simulink model "mCSControls_DG"  (R2012b)
settings: Solver=FixedStepDiscrete  StartTime=0.0  StopTime=10.0  RelTol=1e-3
values from neighbouring files (symbols this model uses):
  CDF2FThreshold = 45    [ControlCal_DG.m]
  CDF2TempThreshold = 20    [ControlCal_DG.m]
  delay = 5    [ControlCal_DG.m]
  DFThresh = 33    [ControlCal_DG.m]
  H = [90 90 90 90]    [ControlCal_DG.m]
  HeatTempThresh1 = 40    [ControlCal_DG.m]
  HeatTempThresh2 = 30    [ControlCal_DG.m]
  HeatTempThresh3 = 20    [ControlCal_DG.m]
  HStabilizationTime = 2*60    (= 120)    [ControlCal_DG.m]
  I_FAN = -1    [ControlCal_DG.m]
  I_VALVE = -1    [ControlCal_DG.m]
  initialSet = [1 1 1]    [ControlCal_DG.m]
  PBFTempThreshold = 30    [ControlCal_DG.m]
  PowerModeSwitchDelay = 30    [ControlCal_DG.m]
  SVocThresh = 550    [ControlCal_DG.m]
  T = [0 4 7 10]    [ControlCal_DG.m]
  Ts = 0.5    [ControlCal_DG.m]
  TSTempSetPoint = -2    [ControlCal_DG.m]
  TV1FThresh = 45    [ControlCal_DG.m]
  TV2FThresh = 60    [ControlCal_DG.m]
  VbatThresh = 22    [ControlCal_DG.m]
  VocDecRate = 0.5    [ControlCal_DG.m]
  VocIncrement = 5    [ControlCal_DG.m]
libraries: c2833xlib x29, simulink x23, c280xlib x11, idelinklib_tgtpref x1
(part 1 of 4)
settings Model: Creator=vinay  LastModifiedBy=vinay
settings DataIOCC: SaveOutput=off  SaveTime=off
settings OptimizationCC: InlineParams=on  UseFloatMulNetSlope=on  UseSpecifiedMinMax=on  InlineInvariantSignals=on  EnhancedBackFolding=on  ZeroExternalMemoryAtStartup=off  NoFixptDivByZeroProtection=on  EfficientFloat2IntCast=on  OptimizeModelRefInitCode=on  LifeSpan=1
settings DebuggingCC: MultiTaskCondExecSysMsg=warning
settings HardwareCC: ProdBitPerChar=16  ProdBitPerInt=16  ProdBitPerPointer=16  ProdLargestAtomicInteger=Integer  ProdIntDivRoundTo=Zero  ProdEndianess=LittleEndian  ProdWordSize=16  ProdHWDeviceType=Texas Instruments->C2000
settings RTWCC: SystemTargetFile=idelink_ert.tlc  GenerateMakefile=off  TemplateMakefile=none  Description=IDE Link ERT  ProcessScript=idelink_ert_make_rtw_hook  CustomInclude=C:\X\DesignFiles\Controls\Gen2\CPUOverrunDetection\  CustomSource=C:\X\DesignFiles\Controls\Gen2\CPUOverrunDetection\CPUOverrunDetection.c  RTWCompilerOptimization=On
settings CodeAppCC: IgnoreCustomStorageClasses=off

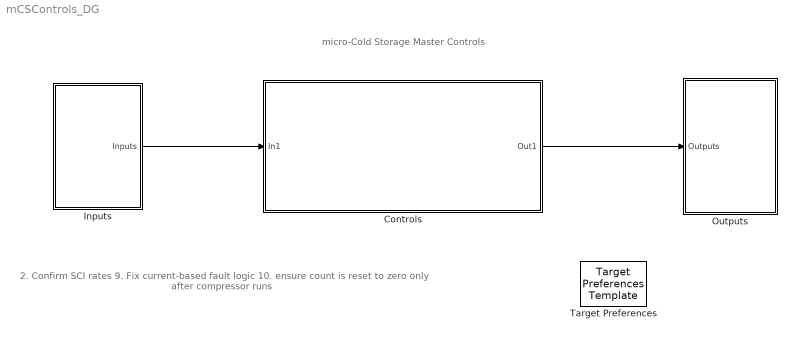
== system mCSControls_DG ==
  note: 2. Confirm SCI rates
      | 9. Fix current-based fault logic
      | 10. ensure count is reset to zero only after compressor runs
  note: micro-Cold Storage Master Controls
  Controls : Subsystem
  Inputs : Subsystem
  Outputs : Subsystem
  Target Preferences : idelinklib_tgtpref/Target Preferences Template  Tag=ccslinktgtpref_ccsv4  library=off
  wires:
  Inputs/1(Inputs) -> Controls/1(In1)
  Controls/1(Out1) -> Outputs/1(Outputs)

== system mCSControls_DG/Controls ==
  In1 : Inport
  Bus Creator : BusCreator  Inputs=2
  Chart : Stateflow chart  TreatAsAtomicUnit=on
  RelayInitialization : Subsystem
  Out1 : Outport
  wires:
  Bus Creator/1 -> Out1/1  "IO"
  In1/1 -> Chart/1(Inputs), Bus Creator/1
  RelayInitialization/1(Relays) -> Chart/2(RelaysOff)
  Chart/1(RelaysOP) -> Bus Creator/2

== system mCSControls_DG/Inputs ==
  Bus Creator : BusCreator  Inputs=6
  DCParams_And_Sensors : Subsystem
  DriveParams : Subsystem
  EEPROM : Subsystem  Commented=on
  HMI : Subsystem
  PowerIP : Subsystem
  Inputs : Outport
  wires:
  Bus Creator/1 -> Inputs/1  "Inputs"
  DCParams_And_Sensors/1(DCParams) -> Bus Creator/1
  DCParams_And_Sensors/2(Sensors) -> Bus Creator/2
  DriveParams/1(DriveParams) -> Bus Creator/3
  HMI/1(HMI) -> Bus Creator/4
  EEPROM/1(EEPROM) -> Bus Creator/5
  PowerIP/1(PowerIP) -> Bus Creator/6

== system mCSControls_DG/Outputs ==
  Outputs : Inport
  DataLogger : Subsystem
  EEPROM : Subsystem  Commented=on
  LCD : Subsystem
  Relays : Subsystem
  wires:
  Outputs/1 -> Relays/1(Inputs), DataLogger/1(Inputs), LCD/1(Inputs), EEPROM/1(Inputs)

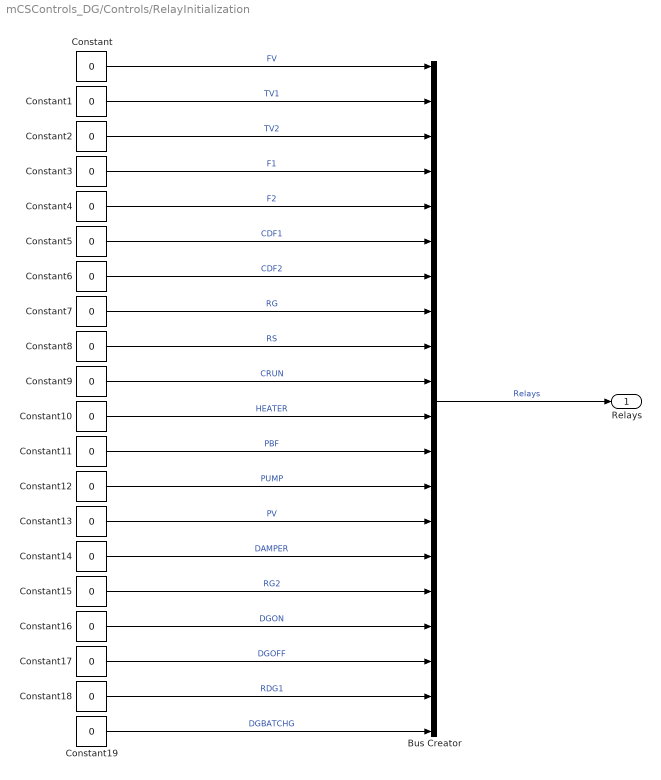
== system mCSControls_DG/Controls/RelayInitialization ==
  Bus Creator : BusCreator  Inputs=20
  Constant{,1..19} (20 alike) : Constant  Value=0  OutDataTypeStr=double
  Relays : Outport
  wires:
  Constant/1 -> Bus Creator/1  "FV"
  Constant13/1 -> Bus Creator/14  "PV"
  Constant12/1 -> Bus Creator/13  "PUMP"
  Constant11/1 -> Bus Creator/12  "PBF"
  Constant10/1 -> Bus Creator/11  "HEATER"
  Constant9/1 -> Bus Creator/10  "CRUN"
  Constant8/1 -> Bus Creator/9  "RS"
  Constant7/1 -> Bus Creator/8  "RG"
  Constant6/1 -> Bus Creator/7  "CDF2"
  Constant5/1 -> Bus Creator/6  "CDF1"
  Constant4/1 -> Bus Creator/5  "F2"
  Constant3/1 -> Bus Creator/4  "F1"
  Constant2/1 -> Bus Creator/3  "TV2"
  Constant1/1 -> Bus Creator/2  "TV1"
  Bus Creator/1 -> Relays/1  "Relays"
  Constant14/1 -> Bus Creator/15  "DAMPER"
  Constant15/1 -> Bus Creator/16  "RG2"
  Constant18/1 -> Bus Creator/19  "RDG1"
  Constant17/1 -> Bus Creator/18  "DGOFF"
  Constant16/1 -> Bus Creator/17  "DGON"
  Constant19/1 -> Bus Creator/20  "DGBATCHG"

== system mCSControls_DG/Inputs/DCParams_And_Sensors ==
  Bus Creator : BusCreator  Inputs=8
  Bus Creator1 : BusCreator  Inputs=9
  Data Type Conversion : DataTypeConversion  OutDataTypeStr=double
  SCI C : c280xlib/SCI Receive  sciModule=C  dataHead=''  dataTail=''  dataType=int16  dataDim=8  initValue=0  errOption=Output the last received value  errValue=0  sampleTime=Ts  outputStatus=off  postInterrupt=off  numFifo=1
  SignalSeperationAndMerging : Subsystem
  DCParams : Outport
  Sensors : Outport  Port=2
  wires:
  SignalSeperationAndMerging/1(Voc) -> Bus Creator/1  "Voc"
  SignalSeperationAndMerging/8(GRID) -> Bus Creator/8  "GRID"
  SignalSeperationAndMerging/2(VBat) -> Bus Creator/2  "Vbat"
  SignalSeperationAndMerging/3(ILoad) -> Bus Creator/3  "Iload"
  SignalSeperationAndMerging/4(IString) -> Bus Creator/4  "Istring"
  SignalSeperationAndMerging/5(F1_HPS) -> Bus Creator/5  "F1_HPS"
  SignalSeperationAndMerging/6(F2_LPS) -> Bus Creator/6  "F2_LPS"
  SignalSeperationAndMerging/7(F3_INT69) -> Bus Creator/7  "F3_INT69"
  Bus Creator/1 -> DCParams/1  "DCParams"
  Bus Creator1/1 -> Sensors/1  "Sensors"
  Data Type Conversion/1 -> SignalSeperationAndMerging/1(Data)
  SignalSeperationAndMerging/9(TH1) -> Bus Creator1/1  "TH1"
  SignalSeperationAndMerging/10(TA) -> Bus Creator1/2  "TA"
  SignalSeperationAndMerging/11(TES1) -> Bus Creator1/3  "TES1"
  SignalSeperationAndMerging/12(TES2) -> Bus Creator1/4  "TES2"
  SignalSeperationAndMerging/13(RH1) -> Bus Creator1/5  "RH1"
  SignalSeperationAndMerging/14(RA) -> Bus Creator1/6  "RA"
  SignalSeperationAndMerging/15(Door) -> Bus Creator1/7  "Door"
  SignalSeperationAndMerging/16(Tank) -> Bus Creator1/8  "Tank"
  SCI C/1 -> Data Type Conversion/1
  SignalSeperationAndMerging/17(Pressure) -> Bus Creator1/9  "Pressure"

== system mCSControls_DG/Inputs/DriveParams ==
  Bus Creator : BusCreator  Inputs=1
  Bus Creator1 : BusCreator  Inputs=3
  Bus Creator2 : BusCreator  Inputs=2
  Demux : Demux
  DriveParamReceive : Subsystem
  From : From  Commented=on  GotoTag=DriveFreq  TagVisibility=global
  Subsystem1 : Subsystem  Commented=on
  DriveParams : Outport
  wires:
  Demux/4 -> Bus Creator/1  "FAULTS"
  Demux/3 -> Bus Creator1/3  "OPCurr"
  Bus Creator1/1 -> Bus Creator2/1  "OP"
  Bus Creator/1 -> Bus Creator2/2  "FAULTS"
  Bus Creator2/1 -> DriveParams/1  "DriveParams"
  DriveParamReceive/1(Data) -> Demux/1
  Demux/1 -> Bus Creator1/1  "OPFreq"
  Demux/2 -> Bus Creator1/2  "OPPower"

== system mCSControls_DG/Inputs/EEPROM ==
  Bus Creator : BusCreator  Inputs=3
  Compare To Zero : simulink/Logic and Bit Operations/Compare To Zero  relop===  OutDataTypeStr=boolean
  Constant : Constant  Value=initialSet
  Data Type Conversion : DataTypeConversion  OutDataTypeStr=double
  Demux : Demux  Outputs=3
  EEPROMRead : Subsystem
  Rate Transition : RateTransition  X0=initialSet  OutPortSampleTime=Ts
  Rate Transition1 : RateTransition  Deterministic=off  OutPortSampleTime=Ts
  Terminator : Terminator
  EEPROM : Outport
  tag scope: Reading=global
  wires:
  Data Type Conversion/1 -> Demux/1
  Demux/1 -> Bus Creator/1  "B"
  Demux/2 -> Bus Creator/2  "M1"
  Demux/3 -> Bus Creator/3  "P1"
  Bus Creator/1 -> EEPROM/1  "EEPROM1"
  Rate Transition/1 -> Data Type Conversion/1
  [Writing] -> Compare To Zero/1
  Compare To Zero/1 -> EEPROMRead/Enable
  EEPROMRead/2(Reading) -> Rate Transition1/1
  Rate Transition1/1 -> [Reading]
  EEPROMRead/1(D) -> Terminator/1
  Constant/1 -> Rate Transition/1

== system mCSControls_DG/Inputs/HMI ==
  Bus Creator : BusCreator  Inputs=3
  Data Detection : MATLAB Function  TreatAsAtomicUnit=on
  Data Type Conversion : DataTypeConversion  OutDataTypeStr=double
  Memory : Memory  X0=initialSet(1)  InheritSampleTime=on
  Memory1 : Memory  X0=initialSet(2)  InheritSampleTime=on
  Memory2 : Memory  X0=initialSet(3)  InheritSampleTime=on
  Rate Transition : RateTransition  Deterministic=off  X0=[250 initialSet 250]
  SCI A Receive : Subsystem
  HMI : Outport
  wires:
  Data Detection/1(B) -> Memory/1, Bus Creator/1  "B"
  Data Detection/2(M1) -> Bus Creator/2, Memory1/1  "M1"
  Data Detection/3(P1) -> Memory2/1, Bus Creator/3  "P1"
  Bus Creator/1 -> HMI/1  "EEPROM"
  Data Type Conversion/1 -> Data Detection/1(u)
  [receiveTrigger] -> SCI A Receive/Trigger
  Memory/1 -> Data Detection/2(Bp)
  Memory1/1 -> Data Detection/3(M1p)
  Memory2/1 -> Data Detection/4(P1p)
  SCI A Receive/1(Out1) -> Rate Transition/1
  Rate Transition/1 -> Data Type Conversion/1

== system mCSControls_DG/Inputs/PowerIP ==
  Bus Creator : BusCreator  Inputs=1
  Constant : Constant  Commented=on
  Data Type Conversion : DataTypeConversion  OutDataTypeStr=double
  Digital Input : c2833xlib/Digital Input  GPIO_Number=GPIO0~GPIO7  GPIO_Bit0=off  GPIO_Bit1=off  GPIO_Bit2=off  GPIO_Bit3=off  GPIO_Bit4=off  GPIO_Bit5=on  GPIO_Bit6=off  GPIO_Bit7=off  sampleTime=Ts  dataType=int16  GPIO_Bit0_Qualification=Sync to SYSCLKOUT  GPIO_Bit1_Qualification=Sync to SYSCLKOUT  GPIO_Bit2_Qualification=Sync to SYSCLKOUT  GPIO_Bit3_Qualification=Sync to SYSCLKOUT  GPIO_Bit4_Qualification=Sync to SYSCLKOUT  GPIO_Bit5_Qualification=Sync to SYSCLKOUT  GPIO_Bit6_Qualification=Sync to SYSCLKOUT  GPIO_Bit7_Qualification=Sync to SYSCLKOUT  Qualification_Period=-1
  Terminator : Terminator  Commented=on
  PowerIP : Outport
  wires:
  Data Type Conversion/1 -> Bus Creator/1  "PowerIP"
  Bus Creator/1 -> PowerIP/1  "PowerIP"
  Digital Input/1 -> Data Type Conversion/1

== system mCSControls_DG/Outputs/DataLogger ==
  Inputs : Inport
  ASCIIAndDataPackaging : Subsystem
  Data Type Conversion1 : DataTypeConversion  Commented=on  OutDataTypeStr=uint8  RndMeth=Simplest
  Debugging : Subsystem  Commented=on
  Rate Transition1 : RateTransition  Deterministic=off  OutPortSampleTime=Tlog
  SCI C : c280xlib/SCI Transmit  sciModule=C  dataHead=''  dataTail=''  postInterrupt=off  numFifo=1
  SCI C1 : c280xlib/SCI Transmit  Commented=on  sciModule=C  dataHead=''  dataTail=''  postInterrupt=off  numFifo=1
  wires:
  ASCIIAndDataPackaging/1(Out1) -> SCI C/1
  Rate Transition1/1 -> ASCIIAndDataPackaging/1(In1)
  Debugging/1(Out1) -> Data Type Conversion1/1
  Data Type Conversion1/1 -> SCI C1/1
  Inputs/1 -> Debugging/1(GUIData), Rate Transition1/1

== system mCSControls_DG/Outputs/EEPROM ==
  Inputs : Inport
  Bus Selector1 : BusSelector  OutputSignals=Inputs.EEPROM  OutputAsBus=on
  ChangeDetection : Subsystem
  OneSecTimer : Stateflow chart  TreatAsAtomicUnit=on
  Subsystem : Subsystem
  tag scope: Writing=global
  wires:
  Inputs/1 -> Bus Selector1/1
  Bus Selector1/1 -> Subsystem/1(D), ChangeDetection/1(D)
  ChangeDetection/1(Change) -> OneSecTimer/1(Input)
  [Reading] -> OneSecTimer/2(Reading)
  OneSecTimer/1(Enable) -> Subsystem/Trigger, [Writing]

== system mCSControls_DG/Outputs/LCD ==
  Inputs : Inport
  Compare To Constant : simulink/Logic and Bit Operations/Compare To Constant  relop===  const=1  OutDataTypeStr=boolean
  Compare To Constant1 : simulink/Logic and Bit Operations/Compare To Constant  relop===  const=2  OutDataTypeStr=boolean
  Compare To Constant2 : simulink/Logic and Bit Operations/Compare To Constant  relop===  const=3  OutDataTypeStr=boolean
  Compare To Constant3 : simulink/Logic and Bit Operations/Compare To Constant  relop===  const=5  OutDataTypeStr=boolean
  DE_RE_One : Subsystem
  DE_RE_Zero : Subsystem
  Rate Transition : RateTransition
  Repeating Sequence Stair : simulink/Sources/Repeating Sequence Stair  OutValues=[1 2 3 4 5].'  tsamp=0.1  OutMin=[]  OutMax=[]  OutDataTypeStr=double  OutputDataTypeScalingMode=double  OutDataType=fixdt(0,8)  ConRadixGroup=Best Precision: Vector-wise  OutScaling=2^-12
  Transmit : Subsystem
  tag scope: receiveTrigger=global
  wires:
  Repeating Sequence Stair/1 -> Compare To Constant3/1, Compare To Constant2/1, Compare To Constant1/1, Compare To Constant/1
  Inputs/1 -> Rate Transition/1
  Compare To Constant2/1 -> DE_RE_Zero/Trigger
  Compare To Constant/1 -> DE_RE_One/Enable
  Compare To Constant1/1 -> Transmit/Trigger
  Rate Transition/1 -> Transmit/1(Inputs)
  Compare To Constant3/1 -> [receiveTrigger]

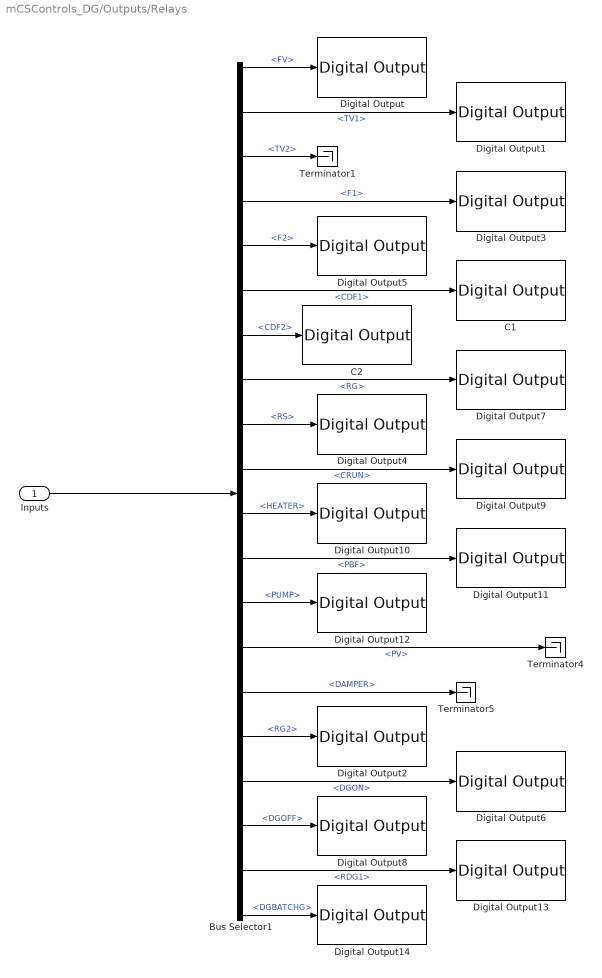
== system mCSControls_DG/Outputs/Relays ==
  Inputs : Inport
  Bus Selector1 : BusSelector  OutputSignals=RelaysOP.FV,RelaysOP.TV1,RelaysOP.TV2,RelaysOP.F1,RelaysOP.F2,RelaysOP.CDF1,RelaysOP.CDF2,RelaysOP.RG,RelaysOP.RS,RelaysOP.CRUN,RelaysOP.HEATER,RelaysOP.PBF,RelaysOP.PUMP,RelaysOP.PV,RelaysOP.DAMPER,RelaysOP.RG2,RelaysOP.DGON,RelaysOP.DGOFF,RelaysOP.RDG1,RelaysOP.DGBATCHG
  C1 : c2833xlib/Digital Output  GPIO_Number=GPIO16~GPIO23  GPIO_Bit0=off  GPIO_BIT0_Toggle=off  GPIO_Bit1=off  GPIO_BIT1_Toggle=off  GPIO_Bit2=off  GPIO_BIT2_Toggle=off  GPIO_Bit3=off  GPIO_BIT3_Toggle=off  GPIO_Bit4=off  GPIO_BIT4_Toggle=off  GPIO_Bit5=off  GPIO_BIT5_Toggle=off  GPIO_Bit6=on  GPIO_BIT6_Toggle=off  GPIO_Bit7=off  GPIO_BIT7_Toggle=off
  C2 : c2833xlib/Digital Output  GPIO_Number=GPIO16~GPIO23  GPIO_Bit0=off  GPIO_BIT0_Toggle=off  GPIO_Bit1=off  GPIO_BIT1_Toggle=off  GPIO_Bit2=off  GPIO_BIT2_Toggle=off  GPIO_Bit3=off  GPIO_BIT3_Toggle=off  GPIO_Bit4=on  GPIO_BIT4_Toggle=off  GPIO_Bit5=off  GPIO_BIT5_Toggle=off  GPIO_Bit6=off  GPIO_BIT6_Toggle=off  GPIO_Bit7=off  GPIO_BIT7_Toggle=off
  Digital Output : c2833xlib/Digital Output  GPIO_Number=GPIO24~GPIO31  GPIO_Bit0=off  GPIO_BIT0_Toggle=off  GPIO_Bit1=off  GPIO_BIT1_Toggle=off  GPIO_Bit2=on  GPIO_BIT2_Toggle=off  GPIO_Bit3=off  GPIO_BIT3_Toggle=off  GPIO_Bit4=off  GPIO_BIT4_Toggle=off  GPIO_Bit5=off  GPIO_BIT5_Toggle=off  GPIO_Bit6=off  GPIO_BIT6_Toggle=off  GPIO_Bit7=off  GPIO_BIT7_Toggle=off
  Digital Output1 : c2833xlib/Digital Output  GPIO_Number=GPIO24~GPIO31  GPIO_Bit0=on  GPIO_BIT0_Toggle=off  GPIO_Bit1=off  GPIO_BIT1_Toggle=off  GPIO_Bit2=off  GPIO_BIT2_Toggle=off  GPIO_Bit3=off  GPIO_BIT3_Toggle=off  GPIO_Bit4=off  GPIO_BIT4_Toggle=off  GPIO_Bit5=off  GPIO_BIT5_Toggle=off  GPIO_Bit6=off  GPIO_BIT6_Toggle=off  GPIO_Bit7=off  GPIO_BIT7_Toggle=off
  Digital Output10 : c2833xlib/Digital Output  GPIO_Number=GPIO80~GPIO87  GPIO_Bit0=off  GPIO_BIT0_Toggle=off  GPIO_Bit1=off  GPIO_BIT1_Toggle=off  GPIO_Bit2=off  GPIO_BIT2_Toggle=off  GPIO_Bit3=off  GPIO_BIT3_Toggle=off  GPIO_Bit4=off  GPIO_BIT4_Toggle=off  GPIO_Bit5=off  GPIO_BIT5_Toggle=off  GPIO_Bit6=on  GPIO_BIT6_Toggle=off  GPIO_Bit7=off  GPIO_BIT7_Toggle=off
  Digital Output11 : c2833xlib/Digital Output  GPIO_Number=GPIO8~GPIO15  GPIO_Bit0=off  GPIO_BIT0_Toggle=off  GPIO_Bit1=off  GPIO_BIT1_Toggle=off  GPIO_Bit2=off  GPIO_BIT2_Toggle=off  GPIO_Bit3=off  GPIO_BIT3_Toggle=off  GPIO_Bit4=off  GPIO_BIT4_Toggle=off  GPIO_Bit5=off  GPIO_BIT5_Toggle=off  GPIO_Bit6=off  GPIO_BIT6_Toggle=off  GPIO_Bit7=on  GPIO_BIT7_Toggle=off
  Digital Output12 : c2833xlib/Digital Output  GPIO_Number=GPIO8~GPIO15  GPIO_Bit0=off  GPIO_BIT0_Toggle=off  GPIO_Bit1=off  GPIO_BIT1_Toggle=off  GPIO_Bit2=off  GPIO_BIT2_Toggle=off  GPIO_Bit3=off  GPIO_BIT3_Toggle=off  GPIO_Bit4=on  GPIO_BIT4_Toggle=off  GPIO_Bit5=off  GPIO_BIT5_Toggle=off  GPIO_Bit6=off  GPIO_BIT6_Toggle=off  GPIO_Bit7=off  GPIO_BIT7_Toggle=off
  Digital Output13 : c2833xlib/Digital Output  GPIO_Number=GPIO16~GPIO23  GPIO_Bit0=off  GPIO_BIT0_Toggle=off  GPIO_Bit1=on  GPIO_BIT1_Toggle=off  GPIO_Bit2=off  GPIO_BIT2_Toggle=off  GPIO_Bit3=off  GPIO_BIT3_Toggle=off  GPIO_Bit4=off  GPIO_BIT4_Toggle=off  GPIO_Bit5=off  GPIO_BIT5_Toggle=off  GPIO_Bit6=off  GPIO_BIT6_Toggle=off  GPIO_Bit7=off  GPIO_BIT7_Toggle=off
  Digital Output14 : c2833xlib/Digital Output  GPIO_Number=GPIO24~GPIO31  GPIO_Bit0=off  GPIO_BIT0_Toggle=off  GPIO_Bit1=off  GPIO_BIT1_Toggle=off  GPIO_Bit2=off  GPIO_BIT2_Toggle=off  GPIO_Bit3=on  GPIO_BIT3_Toggle=off  GPIO_Bit4=off  GPIO_BIT4_Toggle=off  GPIO_Bit5=off  GPIO_BIT5_Toggle=off  GPIO_Bit6=off  GPIO_BIT6_Toggle=off  GPIO_Bit7=off  GPIO_BIT7_Toggle=off
  Digital Output2 : c2833xlib/Digital Output  GPIO_Number=GPIO48~GPIO55  GPIO_Bit0=on  GPIO_BIT0_Toggle=off  GPIO_Bit1=off  GPIO_BIT1_Toggle=off  GPIO_Bit2=off  GPIO_BIT2_Toggle=off  GPIO_Bit3=off  GPIO_BIT3_Toggle=off  GPIO_Bit4=off  GPIO_BIT4_Toggle=off  GPIO_Bit5=off  GPIO_BIT5_Toggle=off  GPIO_Bit6=off  GPIO_BIT6_Toggle=off  GPIO_Bit7=off  GPIO_BIT7_Toggle=off
  Digital Output3 : c2833xlib/Digital Output  GPIO_Number=GPIO16~GPIO23  GPIO_Bit0=off  GPIO_BIT0_Toggle=off  GPIO_Bit1=off  GPIO_BIT1_Toggle=off  GPIO_Bit2=on  GPIO_BIT2_Toggle=off  GPIO_Bit3=off  GPIO_BIT3_Toggle=off  GPIO_Bit4=off  GPIO_BIT4_Toggle=off  GPIO_Bit5=off  GPIO_BIT5_Toggle=off  GPIO_Bit6=off  GPIO_BIT6_Toggle=off  GPIO_Bit7=off  GPIO_BIT7_Toggle=off
  Digital Output4 : c2833xlib/Digital Output  GPIO_Number=GPIO8~GPIO15  GPIO_Bit0=off  GPIO_BIT0_Toggle=off  GPIO_Bit1=off  GPIO_BIT1_Toggle=off  GPIO_Bit2=on  GPIO_BIT2_Toggle=off  GPIO_Bit3=off  GPIO_BIT3_Toggle=off  GPIO_Bit4=off  GPIO_BIT4_Toggle=off  GPIO_Bit5=off  GPIO_BIT5_Toggle=off  GPIO_Bit6=off  GPIO_BIT6_Toggle=off  GPIO_Bit7=off  GPIO_BIT7_Toggle=off
  Digital Output5 : c2833xlib/Digital Output  GPIO_Number=GPIO16~GPIO23  GPIO_Bit0=on  GPIO_BIT0_Toggle=off  GPIO_Bit1=off  GPIO_BIT1_Toggle=off  GPIO_Bit2=off  GPIO_BIT2_Toggle=off  GPIO_Bit3=off  GPIO_BIT3_Toggle=off  GPIO_Bit4=off  GPIO_BIT4_Toggle=off  GPIO_Bit5=off  GPIO_BIT5_Toggle=off  GPIO_Bit6=off  GPIO_BIT6_Toggle=off  GPIO_Bit7=off  GPIO_BIT7_Toggle=off
  Digital Output6 : c2833xlib/Digital Output  GPIO_Number=GPIO16~GPIO23  GPIO_Bit0=off  GPIO_BIT0_Toggle=off  GPIO_Bit1=off  GPIO_BIT1_Toggle=off  GPIO_Bit2=off  GPIO_BIT2_Toggle=off  GPIO_Bit3=off  GPIO_BIT3_Toggle=off  GPIO_Bit4=off  GPIO_BIT4_Toggle=off  GPIO_Bit5=on  GPIO_BIT5_Toggle=off  GPIO_Bit6=off  GPIO_BIT6_Toggle=off  GPIO_Bit7=off  GPIO_BIT7_Toggle=off
  Digital Output7 : c2833xlib/Digital Output  GPIO_Number=GPIO80~GPIO87  GPIO_Bit0=off  GPIO_BIT0_Toggle=off  GPIO_Bit1=off  GPIO_BIT1_Toggle=off  GPIO_Bit2=off  GPIO_BIT2_Toggle=off  GPIO_Bit3=off  GPIO_BIT3_Toggle=off  GPIO_Bit4=on  GPIO_BIT4_Toggle=off  GPIO_Bit5=off  GPIO_BIT5_Toggle=off  GPIO_Bit6=off  GPIO_BIT6_Toggle=off  GPIO_Bit7=off  GPIO_BIT7_Toggle=off
  Digital Output8 : c2833xlib/Digital Output  GPIO_Number=GPIO16~GPIO23  GPIO_Bit0=off  GPIO_BIT0_Toggle=off  GPIO_Bit1=off  GPIO_BIT1_Toggle=off  GPIO_Bit2=off  GPIO_BIT2_Toggle=off  GPIO_Bit3=on  GPIO_BIT3_Toggle=off  GPIO_Bit4=off  GPIO_BIT4_Toggle=off  GPIO_Bit5=off  GPIO_BIT5_Toggle=off  GPIO_Bit6=off  GPIO_BIT6_Toggle=off  GPIO_Bit7=off  GPIO_BIT7_Toggle=off
  Digital Output9 : c2833xlib/Digital Output  GPIO_Number=GPIO8~GPIO15  GPIO_Bit0=on  GPIO_BIT0_Toggle=off  GPIO_Bit1=off  GPIO_BIT1_Toggle=off  GPIO_Bit2=off  GPIO_BIT2_Toggle=off  GPIO_Bit3=off  GPIO_BIT3_Toggle=off  GPIO_Bit4=off  GPIO_BIT4_Toggle=off  GPIO_Bit5=off  GPIO_BIT5_Toggle=off  GPIO_Bit6=off  GPIO_BIT6_Toggle=off  GPIO_Bit7=off  GPIO_BIT7_Toggle=off
  Terminator1 : Terminator
  Terminator4 : Terminator
  Terminator5 : Terminator
  wires:
  Bus Selector1/16 -> Digital Output2/1  "<RG2>"
  Bus Selector1/15 -> Terminator5/1  "<DAMPER>"
  Inputs/1 -> Bus Selector1/1
  Bus Selector1/1 -> Digital Output/1  "<FV>"
  Bus Selector1/2 -> Digital Output1/1  "<TV1>"
  Bus Selector1/3 -> Terminator1/1  "<TV2>"
  Bus Selector1/4 -> Digital Output3/1  "<F1>"
  Bus Selector1/5 -> Digital Output5/1  "<F2>"
  Bus Selector1/6 -> C1/1  "<CDF1>"
  Bus Selector1/7 -> C2/1  "<CDF2>"
  Bus Selector1/8 -> Digital Output7/1  "<RG>"
  Bus Selector1/9 -> Digital Output4/1  "<RS>"
  Bus Selector1/10 -> Digital Output9/1  "<CRUN>"
  Bus Selector1/11 -> Digital Output10/1  "<HEATER>"
  Bus Selector1/12 -> Digital Output11/1  "<PBF>"
  Bus Selector1/13 -> Digital Output12/1  "<PUMP>"
  Bus Selector1/14 -> Terminator4/1  "<PV>"
  Bus Selector1/17 -> Digital Output6/1  "<DGON>"
  Bus Selector1/18 -> Digital Output8/1  "<DGOFF>"
  Bus Selector1/19 -> Digital Output13/1  "<RDG1>"
  Bus Selector1/20 -> Digital Output14/1  "<DGBATCHG>"

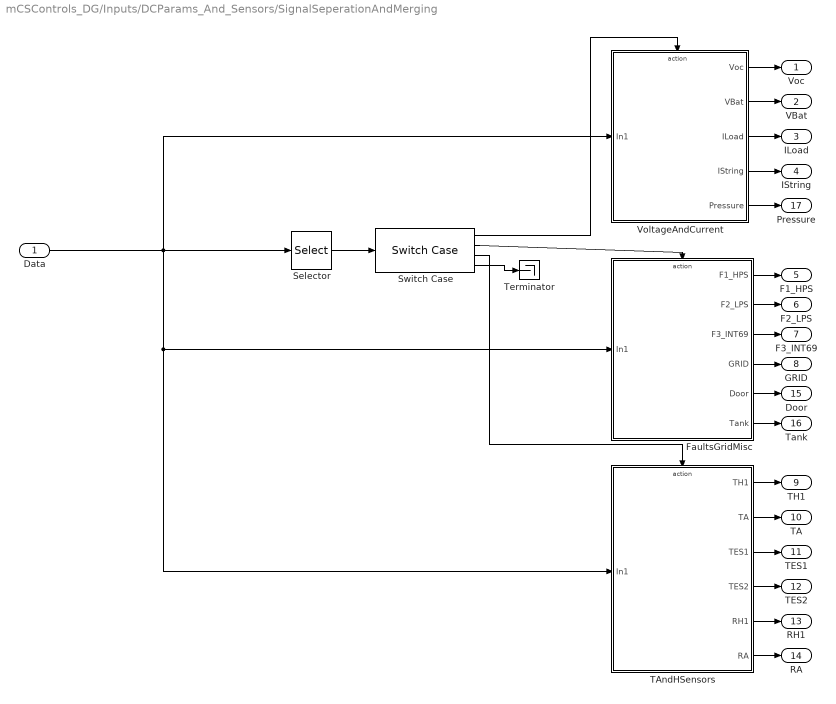
== system mCSControls_DG/Inputs/DCParams_And_Sensors/SignalSeperationAndMerging ==
  Data : Inport
  FaultsGridMisc : Subsystem  TreatAsAtomicUnit=on
  Selector : Selector  InputPortWidth=8  IndexOptions=Index vector (dialog)  Indices=1  OutputSizes=1
  Switch Case : SwitchCase  CaseConditions={1, 2, 3}
  TAndHSensors : Subsystem  TreatAsAtomicUnit=on
  Terminator : Terminator
  VoltageAndCurrent : Subsystem  TreatAsAtomicUnit=on
  Voc : Outport
  VBat : Outport  Port=2
  ILoad : Outport  Port=3
  IString : Outport  Port=4
  F1_HPS : Outport  Port=5
  F2_LPS : Outport  Port=6
  F3_INT69 : Outport  Port=7
  GRID : Outport  Port=8
  TH1 : Outport  Port=9
  TA : Outport  Port=10
  TES1 : Outport  Port=11
  TES2 : Outport  Port=12
  RH1 : Outport  Port=13
  RA : Outport  Port=14
  Door : Outport  Port=15
  Tank : Outport  Port=16
  Pressure : Outport  Port=17
  wires:
  FaultsGridMisc/1(F1_HPS) -> F1_HPS/1
  FaultsGridMisc/2(F2_LPS) -> F2_LPS/1
  VoltageAndCurrent/4(IString) -> IString/1
  FaultsGridMisc/3(F3_INT69) -> F3_INT69/1
  TAndHSensors/2(TA) -> TA/1
  VoltageAndCurrent/2(VBat) -> VBat/1
  TAndHSensors/4(TES2) -> TES2/1
  TAndHSensors/3(TES1) -> TES1/1
  TAndHSensors/1(TH1) -> TH1/1
  TAndHSensors/5(RH1) -> RH1/1
  FaultsGridMisc/4(GRID) -> GRID/1
  TAndHSensors/6(RA) -> RA/1
  VoltageAndCurrent/1(Voc) -> Voc/1
  VoltageAndCurrent/3(ILoad) -> ILoad/1
  Selector/1 -> Switch Case/1
  Data/1 -> TAndHSensors/1(In1), FaultsGridMisc/1(In1), VoltageAndCurrent/1(In1), Selector/1
  Switch Case/1 -> VoltageAndCurrent/Action
  Switch Case/2 -> FaultsGridMisc/Action
  Switch Case/3 -> TAndHSensors/Action
  Switch Case/4 -> Terminator/1
  FaultsGridMisc/5(Door) -> Door/1
  FaultsGridMisc/6(Tank) -> Tank/1
  VoltageAndCurrent/5(Pressure) -> Pressure/1

== system mCSControls_DG/Inputs/DriveParams/DriveParamReceive ==
  Compare To Constant : simulink/Logic and Bit Operations/Compare To Constant  relop===  const=1  OutDataTypeStr=boolean
  Compare To Constant1 : simulink/Logic and Bit Operations/Compare To Constant  relop===  const=2  OutDataTypeStr=boolean
  Compare To Constant2 : simulink/Logic and Bit Operations/Compare To Constant  relop===  const=4  OutDataTypeStr=boolean
  Compare To Constant3 : simulink/Logic and Bit Operations/Compare To Constant  relop===  const=4  OutDataTypeStr=boolean
  DE_RE_One : Subsystem
  IndexIncrement : Subsystem
  Rate Transition1 : RateTransition  Deterministic=off  X0=1
  Repeating Sequence Stair : simulink/Sources/Repeating Sequence Stair  OutValues=[1 2 3 4].'  tsamp=0.5  OutMin=[]  OutMax=[]  OutDataTypeStr=double  OutputDataTypeScalingMode=double  OutDataType=fixdt(0,8)  ConRadixGroup=Best Precision: Vector-wise  OutScaling=2^-12
  Rx : Subsystem
  TxAndDE_RE_Zero : Subsystem
  Data : Outport
  wires:
  Repeating Sequence Stair/1 -> Compare To Constant3/1, Compare To Constant2/1, Compare To Constant1/1, Compare To Constant/1
  Compare To Constant/1 -> DE_RE_One/Enable
  Compare To Constant1/1 -> TxAndDE_RE_Zero/Enable
  Compare To Constant2/1 -> IndexIncrement/Trigger
  IndexIncrement/1(Index) -> [Index]
  [Index] -> Rate Transition1/1
  Rx/1(D) -> Data/1
  Rate Transition1/1 -> TxAndDE_RE_Zero/1(Index)
  [Index] -> Rx/1(Index)
  Compare To Constant3/1 -> Rx/Trigger

== system mCSControls_DG/Inputs/DriveParams/Subsystem1 ==
  note: Freq to Power
  In1 : Inport
  Gain : Gain  Gain=2.72/87
  Out1 : Outport
  wires:
  Gain/1 -> Out1/1
  In1/1 -> Gain/1

== system mCSControls_DG/Inputs/EEPROM/EEPROMRead ==
  Enable : EnablePort
  AddressWrite : Subsystem
  Receive : Subsystem
  Repeating Sequence Stair : simulink/Sources/Repeating Sequence Stair  OutValues=[0 1].'  tsamp=2  OutMin=[]  OutMax=[]  OutDataTypeStr=double  OutputDataTypeScalingMode=double  OutDataType=fixdt(0,8)  ConRadixGroup=Best Precision: Vector-wise  OutScaling=2^-12
  D : Outport
  Reading : Outport  Port=2
  wires:
  Repeating Sequence Stair/1 -> Receive/Trigger, AddressWrite/Trigger, Reading/1
  Receive/1(RD) -> D/1

== system mCSControls_DG/Inputs/HMI/SCI A Receive ==
  Trigger : TriggerPort  TriggerType=falling  PortDimensions=1
  SCI A : c280xlib/SCI Receive  sciModule=A  dataHead=''  dataTail=''  dataType=uint8  dataDim=5  initValue=[250 initialSet 250]  errOption=Output the last received value  errValue=0  sampleTime=-1  outputStatus=off  postInterrupt=off  numFifo=1
  Out1 : Outport
  wires:
  SCI A/1 -> Out1/1

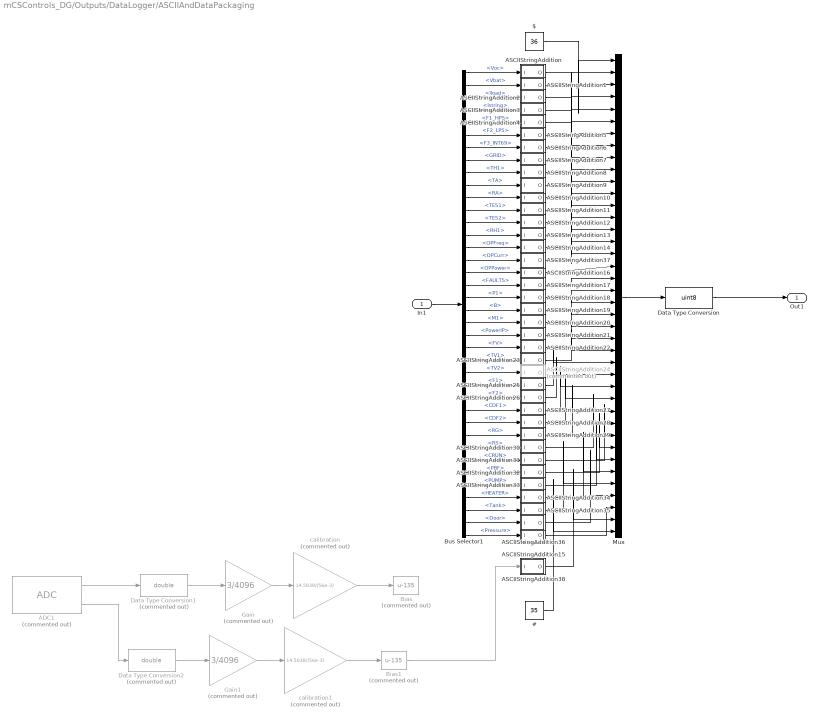
== system mCSControls_DG/Outputs/DataLogger/ASCIIAndDataPackaging ==
  In1 : Inport
  # : Constant  Value=35
  $ : Constant  Value=36
  ADC1 : c280xlib/ADC  Commented=on  useModule=A and B  useMode=Simultaneous  sourceSOC=Software  sourceSOC1=Software  sourceSOC2=Software  xint2_ADCSOC=31  Ts=90  dType=uint16  postInterrupt=off  numConversionsSingle=1  numConversionsDouble=1  conv0=ADCINA0  conv1=ADCINA1  conv2=ADCINA2  conv3=ADCINA3  conv4=ADCINA4  conv5=ADCINA5  conv6=ADCINA6  conv7=ADCINA7  conv8=ADCINB0  conv9=ADCINB1  conv10=ADCINB2  conv11=ADCINB3  conv12=ADCINB4  conv13=ADCINB5  conv14=ADCINB6  conv15=ADCINB7  convAB0=ADCINA3 and ADCINB3  convAB1=ADCINA1 and ADCINB1  convAB2=ADCINA2 and ADCINB2  convAB3=ADCINA3 and ADCINB3  convAB4=ADCINA4 and ADCINB4  convAB5=ADCINA5 and ADCINB5  convAB6=ADCINA6 and ADCINB6  convAB7=ADCINA7 and ADCINB7  convA0=ADCINA3  convA1=ADCINA1  convA2=ADCINA2  convA3=ADCINA3  convA4=ADCINA4  convA5=ADCINA5  convA6=ADCINA6  convA7=ADCINA7  convB0=ADCINB3  convB1=ADCINB1  convB2=ADCINB2  convB3=ADCINB3  convB4=ADCINB4  convB5=ADCINB5  convB6=ADCINB6  convB7=ADCINB7  c28xmultiPort=on  endma=off  chdma=1
  ASCIIStringAddition : Subsystem
  ASCIIStringAddition1 : Subsystem
  ASCIIStringAddition10 : Subsystem
  ASCIIStringAddition11 : Subsystem
  ASCIIStringAddition12 : Subsystem
  ASCIIStringAddition13 : Subsystem
  ASCIIStringAddition14 : Subsystem
  ASCIIStringAddition15 : Subsystem
  ASCIIStringAddition16 : Subsystem
  ASCIIStringAddition17 : Subsystem
  ASCIIStringAddition18 : Subsystem
  ASCIIStringAddition19 : Subsystem
  ASCIIStringAddition2 : Subsystem
  ASCIIStringAddition20 : Subsystem
  ASCIIStringAddition21 : Subsystem
  ASCIIStringAddition22 : Subsystem
  ASCIIStringAddition23 : Subsystem
  ASCIIStringAddition24 : Subsystem  Commented=on
  ASCIIStringAddition25 : Subsystem
  ASCIIStringAddition26 : Subsystem
  ASCIIStringAddition27 : Subsystem
  ASCIIStringAddition28 : Subsystem
  ASCIIStringAddition29 : Subsystem
  ASCIIStringAddition3 : Subsystem
  ASCIIStringAddition30 : Subsystem
  ASCIIStringAddition31 : Subsystem
  ASCIIStringAddition32 : Subsystem
  ASCIIStringAddition33 : Subsystem
  ASCIIStringAddition34 : Subsystem
  ASCIIStringAddition35 : Subsystem
  ASCIIStringAddition36 : Subsystem
  ASCIIStringAddition37 : Subsystem
  ASCIIStringAddition38 : Subsystem
  ASCIIStringAddition4 : Subsystem
  ASCIIStringAddition5 : Subsystem
  ASCIIStringAddition6 : Subsystem
  ASCIIStringAddition7 : Subsystem
  ASCIIStringAddition8 : Subsystem
  ASCIIStringAddition9 : Subsystem
  Bias : Bias  Commented=on  Bias=-135
  Bias1 : Bias  Commented=on  Bias=-135
  Bus Selector1 : BusSelector  OutputSignals=Inputs.DCParams.Voc,Inputs.DCParams.Vbat,Inputs.DCParams.Iload,Inputs.DCParams.Istring,Inputs.DCParams.F1_HPS,Inputs.DCParams.F2_LPS,Inputs.DCParams.F3_INT69,Inputs.DCParams.GRID,Inputs.Sensors.TH1,Inputs.Sensors.TA,Inputs.Sensors.RA,Inputs.Sensors.TES1,Inputs.Sensors.TES2,Inputs.Sensors.RH1,Inputs.DriveParams.OP.OPFreq,Inputs.DriveParams.OP.OPCurr,Inputs.DriveParams.OP.OPPower,Inputs.DriveParams.FAULTS.FAULTS,Inputs.EEPROM.P1,Inputs.EEPROM.B,Inputs.EEPROM.M1,Inputs.PowerIP.PowerIP,RelaysOP.FV,RelaysOP.TV1,RelaysOP.TV2,RelaysOP.F1,RelaysOP.F2,RelaysOP.CDF1,RelaysOP.CDF2,RelaysOP.RG,RelaysOP.RS,RelaysOP.CRUN,RelaysOP.PBF,RelaysOP.PUMP,RelaysOP.HEATER,Inputs.Sensors.Tank,Inputs.Sensors.Door,Inputs.Sensors.Pressure
  Data Type Conversion : DataTypeConversion  OutDataTypeStr=uint8  RndMeth=Simplest
  Data Type Conversion1 : DataTypeConversion  Commented=on  OutDataTypeStr=double
  Data Type Conversion2 : DataTypeConversion  Commented=on  OutDataTypeStr=double
  Gain : Gain  Commented=on  Gain=3/4096
  Gain1 : Gain  Commented=on  Gain=3/4096
  Mux : Mux  Inputs=40
  calibration : Gain  Commented=on  Gain=14.5038/(56e-3)
  calibration1 : Gain  Commented=on  Gain=14.5038/(56e-3)
  Out1 : Outport
  wires:
  Mux/1 -> Data Type Conversion/1
  Data Type Conversion/1 -> Out1/1
  In1/1 -> Bus Selector1/1
  Bus Selector1/16 -> ASCIIStringAddition37/1(I)  "<OPCurr>"
  Bus Selector1/13 -> ASCIIStringAddition12/1(I)  "<TES2>"
  Bus Selector1/19 -> ASCIIStringAddition18/1(I)  "<P1>"
  Bus Selector1/23 -> ASCIIStringAddition22/1(I)  "<FV>"
  Bus Selector1/5 -> ASCIIStringAddition4/1(I)  "<F1_HPS>"
  Bus Selector1/21 -> ASCIIStringAddition20/1(I)  "<M1>"
  Bus Selector1/22 -> ASCIIStringAddition21/1(I)  "<PowerIP>"
  Bus Selector1/4 -> ASCIIStringAddition3/1(I)  "<Istring>"
  Bus Selector1/11 -> ASCIIStringAddition10/1(I)  "<RA>"
  Bus Selector1/14 -> ASCIIStringAddition13/1(I)  "<RH1>"
  Bus Selector1/9 -> ASCIIStringAddition8/1(I)  "<TH1>"
  Bus Selector1/12 -> ASCIIStringAddition11/1(I)  "<TES1>"
  Bus Selector1/20 -> ASCIIStringAddition19/1(I)  "<B>"
  Bus Selector1/17 -> ASCIIStringAddition16/1(I)  "<OPPower>"
  Bus Selector1/18 -> ASCIIStringAddition17/1(I)  "<FAULTS>"
  Bus Selector1/7 -> ASCIIStringAddition6/1(I)  "<F3_INT69>"
  Bus Selector1/1 -> ASCIIStringAddition/1(I)  "<Voc>"
  Bus Selector1/8 -> ASCIIStringAddition7/1(I)  "<GRID>"
  Bus Selector1/6 -> ASCIIStringAddition5/1(I)  "<F2_LPS>"
  Bus Selector1/2 -> ASCIIStringAddition1/1(I)  "<Vbat>"
  Bus Selector1/3 -> ASCIIStringAddition2/1(I)  "<Iload>"
  Bus Selector1/10 -> ASCIIStringAddition9/1(I)  "<TA>"
  Bus Selector1/15 -> ASCIIStringAddition14/1(I)  "<OPFreq>"
  Bus Selector1/24 -> ASCIIStringAddition23/1(I)  "<TV1>"
  Bus Selector1/25 -> ASCIIStringAddition24/1(I)  "<TV2>"
  Bus Selector1/26 -> ASCIIStringAddition25/1(I)  "<F1>"
  Bus Selector1/27 -> ASCIIStringAddition26/1(I)  "<F2>"
  Bus Selector1/28 -> ASCIIStringAddition27/1(I)  "<CDF1>"
  Bus Selector1/34 -> ASCIIStringAddition33/1(I)  "<PUMP>"
  Bus Selector1/35 -> ASCIIStringAddition34/1(I)  "<HEATER>"
  Bus Selector1/29 -> ASCIIStringAddition28/1(I)  "<CDF2>"
  Bus Selector1/30 -> ASCIIStringAddition29/1(I)  "<RG>"
  Bus Selector1/33 -> ASCIIStringAddition32/1(I)  "<PBF>"
  Bus Selector1/31 -> ASCIIStringAddition30/1(I)  "<RS>"
  Bus Selector1/32 -> ASCIIStringAddition31/1(I)  "<CRUN>"
  Bus Selector1/37 -> ASCIIStringAddition36/1(I)  "<Door>"
  Bus Selector1/36 -> ASCIIStringAddition35/1(I)  "<Tank>"
  $/1 -> Mux/1
  ASCIIStringAddition/1(O) -> Mux/2
  ASCIIStringAddition1/1(O) -> Mux/3
  ASCIIStringAddition2/1(O) -> Mux/4
  ASCIIStringAddition3/1(O) -> Mux/5
  ASCIIStringAddition4/1(O) -> Mux/6
  ASCIIStringAddition5/1(O) -> Mux/7
  ASCIIStringAddition6/1(O) -> Mux/8
  ASCIIStringAddition7/1(O) -> Mux/9
  ASCIIStringAddition8/1(O) -> Mux/10
  ASCIIStringAddition9/1(O) -> Mux/11
  ASCIIStringAddition10/1(O) -> Mux/12
  ASCIIStringAddition11/1(O) -> Mux/13
  ASCIIStringAddition12/1(O) -> Mux/14
  ASCIIStringAddition13/1(O) -> Mux/15
  ASCIIStringAddition14/1(O) -> Mux/16
  ASCIIStringAddition37/1(O) -> Mux/17
  ASCIIStringAddition16/1(O) -> Mux/18
  ASCIIStringAddition17/1(O) -> Mux/19
  ASCIIStringAddition18/1(O) -> Mux/20
  ASCIIStringAddition19/1(O) -> Mux/21
  ASCIIStringAddition20/1(O) -> Mux/22
  ASCIIStringAddition21/1(O) -> Mux/23
  ASCIIStringAddition22/1(O) -> Mux/24
  ASCIIStringAddition23/1(O) -> Mux/25
  ASCIIStringAddition25/1(O) -> Mux/26
  Gain/1 -> calibration/1
  calibration/1 -> Bias/1
  Data Type Conversion1/1 -> Gain/1
  ADC1/1 -> Data Type Conversion1/1
  ADC1/2 -> Data Type Conversion2/1
  Data Type Conversion2/1 -> Gain1/1
  Gain1/1 -> calibration1/1
  calibration1/1 -> Bias1/1
  Bias1/1 -> ASCIIStringAddition38/1(I)
  Bus Selector1/38 -> ASCIIStringAddition15/1(I)  "<Pressure>"
  ASCIIStringAddition26/1(O) -> Mux/27
  ASCIIStringAddition27/1(O) -> Mux/28
  ASCIIStringAddition28/1(O) -> Mux/29
  ASCIIStringAddition29/1(O) -> Mux/30
  ASCIIStringAddition30/1(O) -> Mux/31
  ASCIIStringAddition31/1(O) -> Mux/32
  ASCIIStringAddition32/1(O) -> Mux/33
  ASCIIStringAddition33/1(O) -> Mux/34
  ASCIIStringAddition34/1(O) -> Mux/35
  ASCIIStringAddition35/1(O) -> Mux/36
  ASCIIStringAddition36/1(O) -> Mux/37
  ASCIIStringAddition15/1(O) -> Mux/38
  ASCIIStringAddition38/1(O) -> Mux/39
  #/1 -> Mux/40

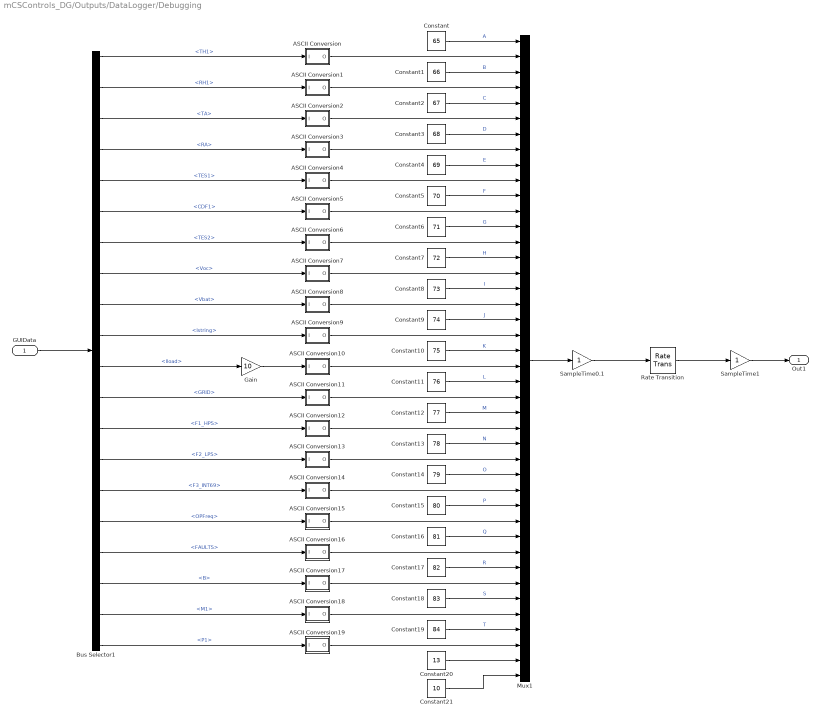
== system mCSControls_DG/Outputs/DataLogger/Debugging ==
  GUIData : Inport
  ASCII Conversion : Subsystem
  ASCII Conversion1 : Subsystem
  ASCII Conversion10 : Subsystem
  ASCII Conversion11 : Subsystem
  ASCII Conversion12 : Subsystem
  ASCII Conversion13 : Subsystem
  ASCII Conversion14 : Subsystem
  ASCII Conversion15 : Subsystem
  ASCII Conversion16 : Subsystem
  ASCII Conversion17 : Subsystem
  ASCII Conversion18 : Subsystem
  ASCII Conversion19 : Subsystem
  ASCII Conversion2 : Subsystem
  ASCII Conversion3 : Subsystem
  ASCII Conversion4 : Subsystem
  ASCII Conversion5 : Subsystem
  ASCII Conversion6 : Subsystem
  ASCII Conversion7 : Subsystem
  ASCII Conversion8 : Subsystem
  ASCII Conversion9 : Subsystem
  Bus Selector1 : BusSelector  OutputSignals=Inputs.Sensors.TH1,Inputs.Sensors.RH1,Inputs.Sensors.TA,Inputs.Sensors.RA,Inputs.Sensors.TES1,RelaysOP.CDF1,Inputs.Sensors.TES2,Inputs.DCParams.Voc,Inputs.DCParams.Vbat,Inputs.DCParams.Istring,Inputs.DCParams.Iload,Inputs.DCParams.GRID,Inputs.DCParams.F1_HPS,Inputs.DCParams.F2_LPS,Inputs.DCParams.F3_INT69,Inputs.DriveParams.OP.OPFreq,Inputs.DriveParams.FAULTS.FAULTS,Inputs.EEPROM1.B,Inputs.EEPROM1.M1,Inputs.EEPROM1.P1
  Constant : Constant  Value=65
  Constant1 : Constant  Value=66
  Constant10 : Constant  Value=75
  Constant11 : Constant  Value=76
  Constant12 : Constant  Value=77
  Constant13 : Constant  Value=78
  Constant14 : Constant  Value=79
  Constant15 : Constant  Value=80
  Constant16 : Constant  Value=81
  Constant17 : Constant  Value=82
  Constant18 : Constant  Value=83
  Constant19 : Constant  Value=84
  Constant2 : Constant  Value=67
  Constant20 : Constant  Value=13
  Constant21 : Constant  Value=10
  Constant3 : Constant  Value=68
  Constant4 : Constant  Value=69
  Constant5 : Constant  Value=70
  Constant6 : Constant  Value=71
  Constant7 : Constant  Value=72
  Constant8 : Constant  Value=73
  Constant9 : Constant  Value=74
  Gain : Gain  Gain=10
  Mux1 : Mux  Inputs=42
  Rate Transition : RateTransition  Deterministic=off
  SampleTime0.1 : Gain  SampleTime=Ts
  SampleTime1 : Gain  SampleTime=1
  Out1 : Outport
  wires:
  Mux1/1 -> SampleTime0.1/1
  SampleTime0.1/1 -> Rate Transition/1
  Rate Transition/1 -> SampleTime1/1
  SampleTime1/1 -> Out1/1
  GUIData/1 -> Bus Selector1/1
  Bus Selector1/2 -> ASCII Conversion1/1(I)  "<RH1>"
  Bus Selector1/3 -> ASCII Conversion2/1(I)  "<TA>"
  Bus Selector1/4 -> ASCII Conversion3/1(I)  "<RA>"
  Bus Selector1/5 -> ASCII Conversion4/1(I)  "<TES1>"
  Bus Selector1/7 -> ASCII Conversion6/1(I)  "<TES2>"
  Bus Selector1/8 -> ASCII Conversion7/1(I)  "<Voc>"
  Bus Selector1/9 -> ASCII Conversion8/1(I)  "<Vbat>"
  Bus Selector1/12 -> ASCII Conversion11/1(I)  "<GRID>"
  Bus Selector1/13 -> ASCII Conversion12/1(I)  "<F1_HPS>"
  Bus Selector1/14 -> ASCII Conversion13/1(I)  "<F2_LPS>"
  Bus Selector1/15 -> ASCII Conversion14/1(I)  "<F3_INT69>"
  Bus Selector1/17 -> ASCII Conversion16/1(I)  "<FAULTS>"
  Constant/1 -> Mux1/1  "A"
  Constant1/1 -> Mux1/3  "B"
  Constant2/1 -> Mux1/5  "C"
  Constant3/1 -> Mux1/7  "D"
  Constant4/1 -> Mux1/9  "E"
  Constant5/1 -> Mux1/11  "F"
  Constant6/1 -> Mux1/13  "G"
  Constant7/1 -> Mux1/15  "H"
  Constant8/1 -> Mux1/17  "I"
  Constant9/1 -> Mux1/19  "J"
  Constant10/1 -> Mux1/21  "K"
  Constant11/1 -> Mux1/23  "L"
  Constant12/1 -> Mux1/25  "M"
  Constant13/1 -> Mux1/27  "N"
  Constant14/1 -> Mux1/29  "O"
  Constant15/1 -> Mux1/31  "P"
  Constant16/1 -> Mux1/33  "Q"
  ASCII Conversion1/1(O) -> Mux1/4
  ASCII Conversion2/1(O) -> Mux1/6
  ASCII Conversion3/1(O) -> Mux1/8
  ASCII Conversion4/1(O) -> Mux1/10
  ASCII Conversion5/1(O) -> Mux1/12
  ASCII Conversion6/1(O) -> Mux1/14
  ASCII Conversion7/1(O) -> Mux1/16
  ASCII Conversion8/1(O) -> Mux1/18
  ASCII Conversion9/1(O) -> Mux1/20
  ASCII Conversion11/1(O) -> Mux1/24
  ASCII Conversion12/1(O) -> Mux1/26
  ASCII Conversion13/1(O) -> Mux1/28
  ASCII Conversion14/1(O) -> Mux1/30
  ASCII Conversion15/1(O) -> Mux1/32
  ASCII Conversion16/1(O) -> Mux1/34
  Bus Selector1/10 -> ASCII Conversion9/1(I)  "<Istring>"
  Bus Selector1/11 -> Gain/1  "<Iload>"
  Constant17/1 -> Mux1/35  "R"
  Constant18/1 -> Mux1/37  "S"
  Constant19/1 -> Mux1/39  "T"
  Bus Selector1/18 -> ASCII Conversion17/1(I)  "<B>"
  Bus Selector1/19 -> ASCII Conversion18/1(I)  "<M1>"
  Bus Selector1/20 -> ASCII Conversion19/1(I)  "<P1>"
  ASCII Conversion17/1(O) -> Mux1/36
  ASCII Conversion18/1(O) -> Mux1/38
  ASCII Conversion19/1(O) -> Mux1/40
  Bus Selector1/6 -> ASCII Conversion5/1(I)  "<CDF1>"
  Constant20/1 -> Mux1/41
  Bus Selector1/1 -> ASCII Conversion/1(I)  "<TH1>"
  ASCII Conversion/1(O) -> Mux1/2
  ASCII Conversion10/1(O) -> Mux1/22
  Gain/1 -> ASCII Conversion10/1(I)
  Constant21/1 -> Mux1/42
  Bus Selector1/16 -> ASCII Conversion15/1(I)  "<OPFreq>"

== system mCSControls_DG/Outputs/EEPROM/ChangeDetection ==
  D : Inport
  Bus Selector : BusSelector  OutputSignals=P1,B,M1
  Compare To Zero : simulink/Logic and Bit Operations/Compare To Zero  relop=~=  OutDataTypeStr=boolean
  Compare To Zero1 : simulink/Logic and Bit Operations/Compare To Zero  relop=~=  OutDataTypeStr=boolean
  Compare To Zero2 : simulink/Logic and Bit Operations/Compare To Zero  relop=~=  OutDataTypeStr=boolean
  Sum : Sum  Inputs=|+-
  Sum1 : Sum  Inputs=|+-
  Sum2 : Sum  Inputs=|+-
  Sum3 : Sum  Inputs=+++
  Unit Delay : UnitDelay  SampleTime=-1
  Unit Delay1 : UnitDelay  SampleTime=-1
  Unit Delay2 : UnitDelay  SampleTime=-1
  Change : Outport
  wires:
  D/1 -> Bus Selector/1
  Bus Selector/1 -> Unit Delay/1, Sum/1  "<P1>"
  Unit Delay/1 -> Sum/2
  Bus Selector/2 -> Sum1/1, Unit Delay1/1  "<B>"
  Unit Delay1/1 -> Sum1/2
  Bus Selector/3 -> Unit Delay2/1, Sum2/1  "<M1>"
  Unit Delay2/1 -> Sum2/2
  Sum3/1 -> Change/1
  Sum/1 -> Compare To Zero/1
  Compare To Zero/1 -> Sum3/1
  Sum1/1 -> Compare To Zero1/1
  Sum2/1 -> Compare To Zero2/1
  Compare To Zero2/1 -> Sum3/3
  Compare To Zero1/1 -> Sum3/2

== system mCSControls_DG/Outputs/EEPROM/Subsystem ==
  D : Inport
  Trigger : TriggerPort  TriggerType=falling  PortDimensions=1
  Bus Selector : BusSelector  OutputSignals=B,M1,P1
  Data Type Conversion : DataTypeConversion  OutDataTypeStr=uint8
  I2C Transmit : c280xlib/I2C Transmit  addrFormat=7-Bit addressing  saSource=Specify via dialog  SAR=80  bitCount=8  STP=on  RM=off  STR=off
  Mux : Mux
  WordAddress : Constant  Value=0  SampleTime=-1
  wires:
  Mux/1 -> Data Type Conversion/1
  Data Type Conversion/1 -> I2C Transmit/1
  D/1 -> Bus Selector/1
  WordAddress/1 -> Mux/1
  Bus Selector/1 -> Mux/2  "<B>"
  Bus Selector/2 -> Mux/3  "<M1>"
  Bus Selector/3 -> Mux/4  "<P1>"

== system mCSControls_DG/Outputs/LCD/DE_RE_One ==
  Enable : EnablePort
  Constant1 : Constant  SampleTime=-1
  Constant2 : Constant  SampleTime=-1
  DE : c2833xlib/Digital Output  GPIO_Number=GPIO16~GPIO23  GPIO_Bit0=off  GPIO_BIT0_Toggle=off  GPIO_Bit1=off  GPIO_BIT1_Toggle=off  GPIO_Bit2=off  GPIO_BIT2_Toggle=off  GPIO_Bit3=off  GPIO_BIT3_Toggle=off  GPIO_Bit4=off  GPIO_BIT4_Toggle=off  GPIO_Bit5=off  GPIO_BIT5_Toggle=off  GPIO_Bit6=off  GPIO_BIT6_Toggle=off  GPIO_Bit7=on  GPIO_BIT7_Toggle=off
  RE : c2833xlib/Digital Output  GPIO_Number=GPIO80~GPIO87  GPIO_Bit0=off  GPIO_BIT0_Toggle=off  GPIO_Bit1=off  GPIO_BIT1_Toggle=off  GPIO_Bit2=off  GPIO_BIT2_Toggle=off  GPIO_Bit3=off  GPIO_BIT3_Toggle=off  GPIO_Bit4=off  GPIO_BIT4_Toggle=off  GPIO_Bit5=off  GPIO_BIT5_Toggle=off  GPIO_Bit6=off  GPIO_BIT6_Toggle=off  GPIO_Bit7=on  GPIO_BIT7_Toggle=off
  wires:
  Constant1/1 -> DE/1
  Constant2/1 -> RE/1

== system mCSControls_DG/Outputs/LCD/DE_RE_Zero ==
  Trigger : TriggerPort  PortDimensions=1
  Constant1 : Constant  Value=0  SampleTime=-1
  Constant2 : Constant  Value=0  SampleTime=-1
  DE : c2833xlib/Digital Output  GPIO_Number=GPIO16~GPIO23  GPIO_Bit0=off  GPIO_BIT0_Toggle=off  GPIO_Bit1=off  GPIO_BIT1_Toggle=off  GPIO_Bit2=off  GPIO_BIT2_Toggle=off  GPIO_Bit3=off  GPIO_BIT3_Toggle=off  GPIO_Bit4=off  GPIO_BIT4_Toggle=off  GPIO_Bit5=off  GPIO_BIT5_Toggle=off  GPIO_Bit6=off  GPIO_BIT6_Toggle=off  GPIO_Bit7=on  GPIO_BIT7_Toggle=off
  RE : c2833xlib/Digital Output  GPIO_Number=GPIO80~GPIO87  GPIO_Bit0=off  GPIO_BIT0_Toggle=off  GPIO_Bit1=off  GPIO_BIT1_Toggle=off  GPIO_Bit2=off  GPIO_BIT2_Toggle=off  GPIO_Bit3=off  GPIO_BIT3_Toggle=off  GPIO_Bit4=off  GPIO_BIT4_Toggle=off  GPIO_Bit5=off  GPIO_BIT5_Toggle=off  GPIO_Bit6=off  GPIO_BIT6_Toggle=off  GPIO_Bit7=on  GPIO_BIT7_Toggle=off
  wires:
  Constant2/1 -> RE/1
  Constant1/1 -> DE/1

== system mCSControls_DG/Outputs/LCD/Transmit ==
  Inputs : Inport
  Trigger : TriggerPort  PortDimensions=1
  Bus Selector : BusSelector  OutputSignals=Inputs.EEPROM.B,Inputs.EEPROM.M1,Inputs.EEPROM.P1,Inputs.Sensors.TH1,Inputs.Sensors.RH1,Inputs.DriveParams.OP.OPPower
  Constant : Constant  Value=255
  Constant1 : Constant  Value=254
  Constant2 : Constant  Value=253
  Data Type Conversion : DataTypeConversion  OutDataTypeStr=uint8
  Gain : Gain  Gain=10
  LEDOnPanelBox : Subsystem  Commented=on
  Mux : Mux  Inputs=10
  SCI A : c280xlib/SCI Transmit  sciModule=A  dataHead=''  dataTail=''  postInterrupt=off  numFifo=1
  SetpointAchieved : Subsystem
  wires:
  SetpointAchieved/1(LED) -> Mux/10, LEDOnPanelBox/2(TH1Achieved)
  Bus Selector/4 -> Mux/7, SetpointAchieved/1(TH1)  "<TH1>"
  Bus Selector/2 -> SetpointAchieved/2(B), Mux/5  "<M1>"
  Bus Selector/6 -> Gain/1  "<OPPower>"
  Bus Selector/1 -> LEDOnPanelBox/1(P), Mux/4  "<B>"
  Inputs/1 -> Bus Selector/1
  Mux/1 -> Data Type Conversion/1
  Data Type Conversion/1 -> SCI A/1
  Constant/1 -> Mux/1
  Constant1/1 -> Mux/2
  Constant2/1 -> Mux/3
  Bus Selector/3 -> Mux/6  "<P1>"
  Bus Selector/5 -> Mux/8  "<RH1>"
  Gain/1 -> Mux/9

== system mCSControls_DG/Inputs/DCParams_And_Sensors/SignalSeperationAndMerging/FaultsGridMisc ==
  In1 : Inport
  Action Port : ActionPort  ActionType=case
  Demux : Demux  Outputs=8
  Gain{1..6} (6 alike) : Gain  Gain=0.1
  Terminator : Terminator
  Terminator3 : Terminator
  F1_HPS : Outport  InitialOutput=0
  F2_LPS : Outport  Port=2  InitialOutput=0
  F3_INT69 : Outport  Port=3  InitialOutput=0
  GRID : Outport  Port=4  InitialOutput=0
  Door : Outport  Port=5  InitialOutput=0
  Tank : Outport  Port=6  InitialOutput=0
  wires:
  Demux/8 -> Terminator3/1
  Demux/7 -> Gain6/1
  Demux/6 -> Gain5/1
  Demux/1 -> Terminator/1
  Demux/5 -> Gain4/1
  Demux/4 -> Gain2/1
  Demux/3 -> Gain1/1
  Demux/2 -> Gain3/1
  In1/1 -> Demux/1
  Gain3/1 -> F1_HPS/1
  Gain1/1 -> F2_LPS/1
  Gain2/1 -> F3_INT69/1
  Gain4/1 -> GRID/1
  Gain5/1 -> Door/1
  Gain6/1 -> Tank/1

== system mCSControls_DG/Inputs/DCParams_And_Sensors/SignalSeperationAndMerging/TAndHSensors ==
  note: As sensor is placed in a very hot position - through experimentation, it is observed average room temperature is 3 degrees cooler
  In1 : Inport
  Action Port : ActionPort  ActionType=case
  Bias : Bias  Bias=-3
  Demux : Demux  Outputs=8
  Gain{1..6} (6 alike) : Gain  Gain=0.1
  Terminator : Terminator
  Terminator1 : Terminator
  TH1 : Outport  InitialOutput=0
  TA : Outport  Port=2  InitialOutput=0
  TES1 : Outport  Port=3  InitialOutput=0
  TES2 : Outport  Port=4  InitialOutput=0
  RH1 : Outport  Port=5  InitialOutput=0
  RA : Outport  Port=6  InitialOutput=0
  wires:
  In1/1 -> Demux/1
  Demux/2 -> Gain3/1
  Demux/3 -> Gain1/1
  Demux/4 -> Gain2/1
  Demux/5 -> Gain4/1
  Demux/1 -> Terminator/1
  Demux/6 -> Gain5/1
  Demux/7 -> Gain6/1
  Demux/8 -> Terminator1/1
  Gain1/1 -> TA/1
  Gain2/1 -> TES1/1
  Gain4/1 -> TES2/1
  Gain5/1 -> RH1/1
  Gain6/1 -> RA/1
  Gain3/1 -> Bias/1
  Bias/1 -> TH1/1

== system mCSControls_DG/Inputs/DCParams_And_Sensors/SignalSeperationAndMerging/VoltageAndCurrent ==
  In1 : Inport
  Action Port : ActionPort  ActionType=case
  Bias : Bias  Bias=-10
  Bias1 : Bias  Bias=-10
  Demux : Demux  Outputs=8
  Gain{,1..4} (5 alike) : Gain  Gain=0.1
  Terminator : Terminator
  Terminator2 : Terminator
  Terminator3 : Terminator
  Voc : Outport  InitialOutput=0
  VBat : Outport  Port=2  InitialOutput=0
  ILoad : Outport  Port=3  InitialOutput=0
  IString : Outport  Port=4  InitialOutput=0
  Pressure : Outport  Port=5  InitialOutput=0
  wires:
  In1/1 -> Demux/1
  Demux/2 -> Gain/1
  Demux/3 -> Gain1/1
  Demux/4 -> Gain2/1
  Demux/5 -> Gain3/1
  Demux/1 -> Terminator/1
  Demux/6 -> Gain4/1
  Demux/7 -> Terminator2/1
  Demux/8 -> Terminator3/1
  Gain/1 -> Voc/1
  Gain1/1 -> VBat/1
  Gain2/1 -> Bias/1
  Gain3/1 -> Bias1/1
  Bias/1 -> ILoad/1
  Gain4/1 -> Pressure/1
  Bias1/1 -> IString/1

== system mCSControls_DG/Inputs/DriveParams/DriveParamReceive/DE_RE_One ==
  Enable : EnablePort
  DE : Constant  SampleTime=-1
  Digital Output : c2833xlib/Digital Output  GPIO_Number=GPIO0~GPIO7  GPIO_Bit0=off  GPIO_BIT0_Toggle=off  GPIO_Bit1=off  GPIO_BIT1_Toggle=off  GPIO_Bit2=off  GPIO_BIT2_Toggle=off  GPIO_Bit3=off  GPIO_BIT3_Toggle=off  GPIO_Bit4=off  GPIO_BIT4_Toggle=off  GPIO_Bit5=off  GPIO_BIT5_Toggle=off  GPIO_Bit6=off  GPIO_BIT6_Toggle=off  GPIO_Bit7=on  GPIO_BIT7_Toggle=off
  Digital Output1 : c2833xlib/Digital Output  GPIO_Number=GPIO48~GPIO55  GPIO_Bit0=off  GPIO_BIT0_Toggle=off  GPIO_Bit1=on  GPIO_BIT1_Toggle=off  GPIO_Bit2=off  GPIO_BIT2_Toggle=off  GPIO_Bit3=off  GPIO_BIT3_Toggle=off  GPIO_Bit4=off  GPIO_BIT4_Toggle=off  GPIO_Bit5=off  GPIO_BIT5_Toggle=off  GPIO_Bit6=off  GPIO_BIT6_Toggle=off  GPIO_Bit7=off  GPIO_BIT7_Toggle=off
  RE : Constant  Value=0  SampleTime=-1
  wires:
  DE/1 -> Digital Output/1
  RE/1 -> Digital Output1/1

== system mCSControls_DG/Inputs/DriveParams/DriveParamReceive/IndexIncrement ==
  Trigger : TriggerPort  TriggerType=falling  PortDimensions=1
  Add : Sum
  Bias : Bias  Bias=1
  Constant : Constant
  Constant1 : Constant  Value=4
  Math Function : Math  Operator=rem  SaturateOnIntegerOverflow=on
  Memory : Memory  InheritSampleTime=on
  Index : Outport  InitialOutput=1
  wires:
  Constant/1 -> Add/1
  Add/1 -> Math Function/1
  Constant1/1 -> Math Function/2
  Memory/1 -> Add/2
  Math Function/1 -> Bias/1, Memory/1
  Bias/1 -> Index/1

== system mCSControls_DG/Inputs/DriveParams/DriveParamReceive/Rx ==
  Index : Inport
  Trigger : TriggerPort  PortDimensions=1
  Compare To Constant : simulink/Logic and Bit Operations/Compare To Constant  relop===  const=1  OutDataTypeStr=boolean
  Compare To Constant1 : simulink/Logic and Bit Operations/Compare To Constant  relop===  const=2  OutDataTypeStr=boolean
  Compare To Constant2 : simulink/Logic and Bit Operations/Compare To Constant  relop===  const=3  OutDataTypeStr=boolean
  Compare To Constant3 : simulink/Logic and Bit Operations/Compare To Constant  relop===  const=4  OutDataTypeStr=boolean
  FAULTSRx : Subsystem
  Mux : Mux
  OPCurrRx : Subsystem
  OPFreqRx : Subsystem
  OPPowerRx : Subsystem
  SCI B Receive : c280xlib/SCI Receive  sciModule=B  dataHead=''  dataTail=''  dataType=uint8  dataDim=15  initValue=0  errOption=Output custom value  errValue=0  sampleTime=-1  outputStatus=off  postInterrupt=off  numFifo=1
  D : Outport
  wires:
  Compare To Constant/1 -> OPFreqRx/Enable
  Compare To Constant1/1 -> OPPowerRx/Enable
  Compare To Constant2/1 -> OPCurrRx/Enable
  Compare To Constant3/1 -> FAULTSRx/Enable
  Index/1 -> Compare To Constant1/1, Compare To Constant3/1, Compare To Constant2/1, Compare To Constant/1
  OPFreqRx/1(D) -> Mux/1
  OPPowerRx/1(D) -> Mux/2
  OPCurrRx/1(D) -> Mux/3
  FAULTSRx/1(D) -> Mux/4
  SCI B Receive/1 -> OPPowerRx/1(SCIBRx), OPFreqRx/1(SCIBRx), FAULTSRx/1(SCIBRx), OPCurrRx/1(SCIBRx)
  Mux/1 -> D/1

== system mCSControls_DG/Inputs/DriveParams/DriveParamReceive/TxAndDE_RE_Zero ==
  Index : Inport
  Enable : EnablePort  StatesWhenEnabling=reset
  DE_RE_Zero : Subsystem
  FAULTSTx : Subsystem
  Multiport Switch : MultiPortSwitch  Inputs=4
  OPCurrTx : Subsystem
  OPFreqTx : Subsystem
  OPPowerTx : Subsystem
  Repeating Sequence Stair : simulink/Sources/Repeating Sequence Stair  OutValues=[1 0 0 0 0 0].'  tsamp=0.1  OutMin=[]  OutMax=[]  OutDataTypeStr=double  OutputDataTypeScalingMode=double  OutDataType=fixdt(0,8)  ConRadixGroup=Best Precision: Vector-wise  OutScaling=2^-12
  SCI B Tx : Subsystem
  wires:
  Repeating Sequence Stair/1 -> SCI B Tx/Trigger, DE_RE_Zero/Trigger
  Multiport Switch/1 -> SCI B Tx/1(In1)
  Index/1 -> Multiport Switch/1
  OPFreqTx/1(SCIBTx) -> Multiport Switch/2
  OPPowerTx/1(SCIBTx) -> Multiport Switch/3
  OPCurrTx/1(SCIBTx) -> Multiport Switch/4
  FAULTSTx/1(SCIBTx) -> Multiport Switch/5
